simulink model "Parent"  (R2023a)
settings: Solver=FixedStepAuto  StartTime=0.0  StopTime=10.0  RelTol=1e-3
undefined symbols (not defined in the file): RGB
libraries: androidcommunicationlib x4, androidaudiovideolib x2, androiduilib x2
settings Model: Creator=Abhishek  LastModifiedBy=agarw_crynhxp
settings OptimizationCC: EnhancedBackFolding=on  PassReuseOutputArgsThreshold=0  MaxStackSize=64  OptimizeBlockOrder=speed  DifferentSizesBufferReuse=on  OptimizationCustomize=off
settings DebuggingCC: ParameterTunabilityLossMsg=error
settings HardwareCC: ProdBitPerPointer=32  ProdBitPerSizeT=32  ProdBitPerPtrDiffT=32  ProdLargestAtomicInteger=Long  ProdLargestAtomicFloat=Double  ProdWordSize=32  ProdHWDeviceType=ARM Compatible->ARM Cortex  UseEmbeddedCoderFeatures=off  UseSimulinkCoderFeatures=off
settings SFSimCC: MATLABDynamicMemAlloc=off
settings RTWCC: Description=Embedded Coder  SystemTargetFile=ert.tlc  HardwareBoard=Android Device  TLCOptions="-aInlineSetEventsForThisBaseRateFcn=TLC_FALSE -aSuppressMultiTaskScheduler=TLC_FALSE  -aRateBasedStepFcn=0"  TemplateMakefile=ert_default_tmf  RTWVerbose=off  Toolchain=Android SDK/NDK Tools
settings CodeAppCC: ForceParamTrailComments=on  OperatorAnnotations=on
settings ERTTargetCC: ERTCustomFileBanners=off  SupportContinuousTime=on  SupportNonInlinedSFcns=on  RemoveResetFunc=off  ModelStepFunctionPrototypeControlCompliant=off

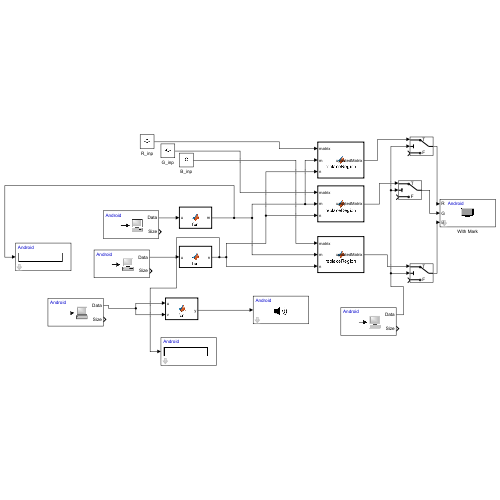
[thumbnail: Simulink's stored preview of the top-level diagram]
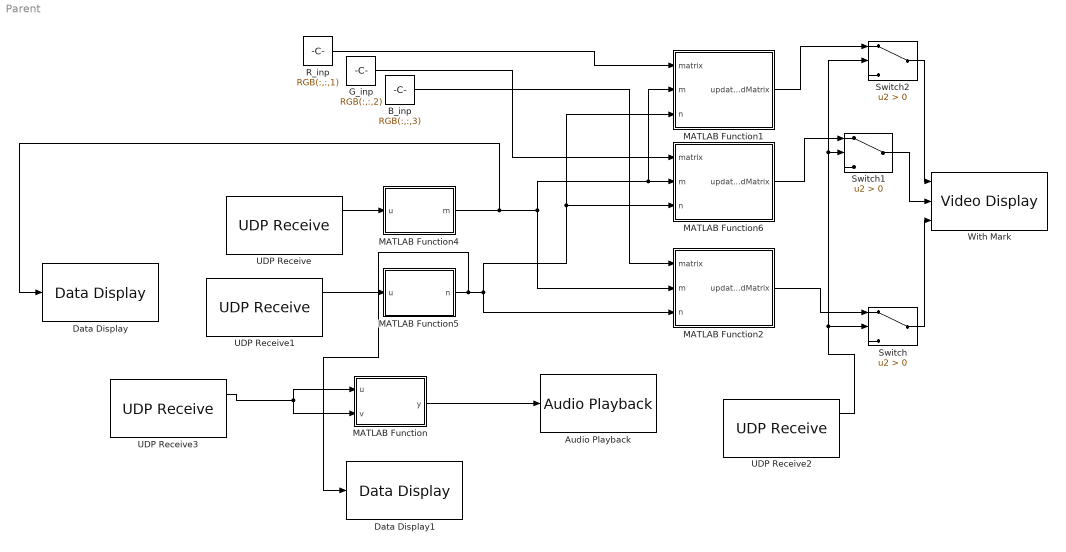
== system Parent ==
  Audio Playback : androidaudiovideolib/Audio Playback  SampleFreq=24000  AudioSamplingFreq=24000  SampleTime=0.1  DeviceStr=0  QueueDuration=0  BlockPlatform=Android
  B_inp : Constant  Value=RGB(:,:,3)  VectorParams1D=off  OutDataTypeStr=Inherit: Inherit via back propagation
  Data Display : androiduilib/Data Display  DataDisplayId=Parent/Data_Display  Format=Float  Precision=6  SimulateUsing=Code generation  blockPlatform=Android
  Data Display1 : androiduilib/Data Display  DataDisplayId=Parent/Data_Display1  Format=Float  Precision=6  SimulateUsing=Code generation  blockPlatform=Android
  G_inp : Constant  Value=RGB(:,:,2)  VectorParams1D=off
  MATLAB Function : MATLAB Function  TreatAsAtomicUnit=on
  MATLAB Function1 : MATLAB Function  TreatAsAtomicUnit=on
  MATLAB Function2 : MATLAB Function  TreatAsAtomicUnit=on
  MATLAB Function4 : MATLAB Function  TreatAsAtomicUnit=on
  MATLAB Function5 : MATLAB Function  TreatAsAtomicUnit=on
  MATLAB Function6 : MATLAB Function  TreatAsAtomicUnit=on
  R_inp : Constant  Value=RGB(:,:,1)  VectorParams1D=off
  Switch : Switch  Criteria=u2 > Threshold  SaturateOnIntegerOverflow=off  InputSameDT=off
  Switch1 : Switch  Criteria=u2 > Threshold  SaturateOnIntegerOverflow=off  InputSameDT=off
  Switch2 : Switch  Criteria=u2 > Threshold  SaturateOnIntegerOverflow=off  InputSameDT=off
  UDP Receive : androidcommunicationlib/UDP Receive  localURL='0.0.0.0'  localPort=25114  remoteURL='0.0.0.0'  remotePort=-1  recvBufferSize=8192  signalDatatype=double  dims=1  isVarSize=off  showBlockingTime=off  blockingTime=0  sampletime=0.1  blockPlatform=Android
  UDP Receive1 : androidcommunicationlib/UDP Receive  localURL='0.0.0.0'  localPort=25113  remoteURL='0.0.0.0'  remotePort=-1  recvBufferSize=8192  signalDatatype=double  dims=1  isVarSize=off  showBlockingTime=off  blockingTime=0  sampletime=0.1  blockPlatform=Android
  UDP Receive2 : androidcommunicationlib/UDP Receive  localURL='0.0.0.0'  localPort=25112  remoteURL='0.0.0.0'  remotePort=-1  recvBufferSize=8192  signalDatatype=boolean  dims=1  isVarSize=off  showBlockingTime=off  blockingTime=0  sampletime=0.5  blockPlatform=Android
  UDP Receive3 : androidcommunicationlib/UDP Receive  localURL='0.0.0.0'  localPort=25111  remoteURL='0.0.0.0'  remotePort=-1  recvBufferSize=8192  signalDatatype=int16  dims=2400  isVarSize=off  showBlockingTime=off  blockingTime=0  sampletime=0.1  blockPlatform=Android
  With Mark : androidaudiovideolib/Video Display  BlockPlatform=Android
  wires:
  MATLAB Function5/1(n) -> Data Display1/1, MATLAB Function1/3(n), MATLAB Function6/3(n), MATLAB Function2/3(n)
  G_inp/1 -> MATLAB Function6/1(matrix)
  B_inp/1 -> MATLAB Function2/1(matrix)
  UDP Receive/1 -> MATLAB Function4/1(u)
  UDP Receive1/1 -> MATLAB Function5/1(u)
  R_inp/1 -> MATLAB Function1/1(matrix)
  UDP Receive3/1 -> MATLAB Function/1(u), MATLAB Function/2(v)
  MATLAB Function/1(y) -> Audio Playback/1
  MATLAB Function1/1(updatedMatrix) -> Switch2/1
  Switch2/1 -> With Mark/1
  MATLAB Function6/1(updatedMatrix) -> Switch1/1
  Switch1/1 -> With Mark/2
  MATLAB Function2/1(updatedMatrix) -> Switch/1
  Switch/1 -> With Mark/3
  UDP Receive2/1 -> Switch/2, Switch1/2, Switch2/2
  MATLAB Function4/1(m) -> Data Display/1, MATLAB Function1/2(m), MATLAB Function6/2(m), MATLAB Function2/2(m)

== matlab function Parent/MATLAB Function1 ==
  data: updatedMatrix output; matrix input; m input; n input
function updatedMatrix = replaceRegion(matrix, m, n)
    [rows, cols] = size(matrix);
    if m < 7 || m > rows - 7 ||  n < 7 || n > cols - 7
        error('Invalid values for m and n. They should be at least 7 and within matrix dimensions - 7.');
    end
    
    updatedMatrix = matrix;

    rowStart = m - 7;
    rowEnd = m + 7;
    colStart = n - 7;
    colEnd = n + 7;

    rowStart = max(1, rowStart);
    rowEnd = min(rows, rowEnd);
    colStart = max(1, colStart);
    colEnd = min(cols, colEnd);

    updatedMatrix(rowStart:rowEnd, colStart:colEnd) = 0;
end

== matlab function Parent/MATLAB Function2 ==
  data: updatedMatrix output; matrix input; m input; n input
function updatedMatrix = replaceRegion(matrix, m, n)
    [rows, cols] = size(matrix);
    if m < 7 || m > rows - 7 || n < 7 || n > cols - 7
        error('Invalid values for m and n. They should be at least 7 and within matrix dimensions - 7.');
    end
    
    updatedMatrix = matrix;

    rowStart = m - 7;
    rowEnd = m + 7;
    colStart = n - 7;
    colEnd = n + 7;

    rowStart = max(1, rowStart);
    rowEnd = min(rows, rowEnd);
    colStart = max(1, colStart);
    colEnd = min(cols, colEnd);

    updatedMatrix(rowStart:rowEnd, colStart:colEnd) = 255;
end

== matlab function Parent/MATLAB Function4 ==
  data: u input; m output
function m = fcn(u)
    a=2.539640591966173e-6;
    md = (23.213259-u)/a;
    m = int16(md);

== matlab function Parent/MATLAB Function5 ==
  data: u input; n output
function n = fcn(u)
    b=3.72962962962963e-6;
    nd = (72.686553-u)/b;
    n = int16(nd);

== matlab function Parent/MATLAB Function ==
  data: u input; y output; v input
function y = fcn(u,v)
    y=[u,v];

end

== matlab function Parent/MATLAB Function6 ==
  data: updatedMatrix output; matrix input; m input; n input
function updatedMatrix = replaceRegion(matrix, m, n)
    [rows, cols] = size(matrix);
    if m < 7 || m > rows - 7 ||  n < 7 || n > cols - 7
        error('Invalid values for m and n. They should be at least 7 and within matrix dimensions - 7.');
    end
 
    updatedMatrix = matrix;

    rowStart = m - 7;
    rowEnd = m + 7;
    colStart = n - 7;
    colEnd = n + 7;

    rowStart = max(1, rowStart);
    rowEnd = min(rows, rowEnd);
    colStart = max(1, colStart);
    colEnd = min(cols, colEnd);

    updatedMatrix(rowStart:rowEnd, colStart:colEnd) = 0;
end
